simulink model "velo_pi"  (Simulink 7.9)
settings: Solver=ode4  StartTime=0.0  StopTime=20  RelTol=1e-3
values from neighbouring files (symbols this model uses):
  ts = 1/50    (= 0.02)    [velo_id_gain.m]    (also in velo_id_tc.m; velo_pi_mbd.m)
libraries: arduino_io_lib x5, simulink x1
settings Model: Creator=hirata  LastModifiedBy=hirata

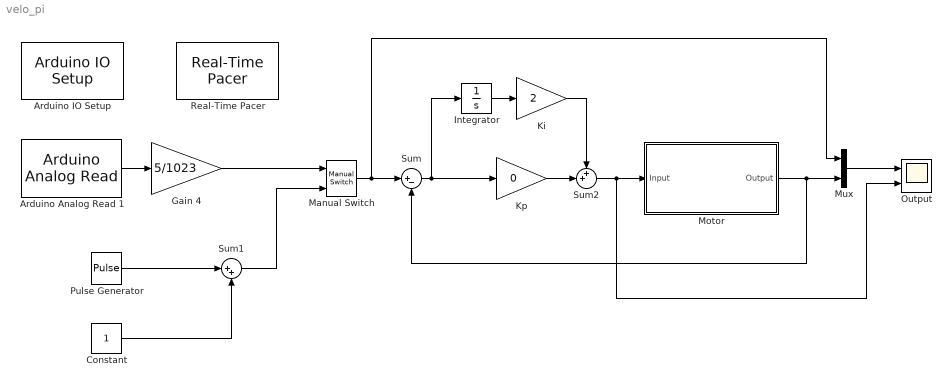
== system velo_pi ==
  Arduino Analog Read 1 : arduino_io_lib/Arduino Analog Read  arduinoVar=Temporary arduino variable: Arduino1  arduinoPin=1  T=ts
  Arduino IO Setup : arduino_io_lib/Arduino IO Setup  Priority=3  arduinoVar=Temporary arduino variable: Arduino1  workspaceVarName=a  comPort=COM3
  Constant : Constant
  Gain 4 : Gain  Gain=5/1023
  Integrator : Integrator
  Ki : Gain  Gain=2
  Kp : Gain  Gain=0
  Manual Switch : simulink/Signal Routing/Manual Switch  sw=0  action=0  varsize=off
  Motor : Subsystem
  Mux : Mux  Inputs=2
  Output : Scope  NumInputPorts=2
      settings: TimeRange=10  YMin=0~0  YMax=2~5
  Pulse Generator : DiscretePulseGenerator  Amplitude=0.5  Period=10/ts  PulseWidth=5/ts  SampleTime=ts
  Real-Time Pacer : arduino_io_lib/Real-Time Pacer  simTimePerRealTime=1
  Sum : Sum  Inputs=|+-
  Sum1 : Sum  Inputs=|++
  Sum2 : Sum  Inputs=++|
  wires:
  Motor/1(Output) -> Mux/2, Sum/2
  Mux/1 -> Output/1
  Arduino Analog Read 1/1 -> Gain 4/1
  Sum2/1 -> Motor/1(Input), Output/2
  Sum/1 -> Kp/1, Integrator/1
  Manual Switch/1 -> Sum/1, Mux/1
  Gain 4/1 -> Manual Switch/1
  Constant/1 -> Sum1/2
  Pulse Generator/1 -> Sum1/1
  Sum1/1 -> Manual Switch/2
  Integrator/1 -> Ki/1
  Ki/1 -> Sum2/1
  Kp/1 -> Sum2/2

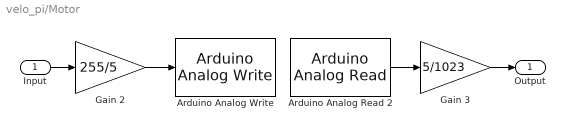
== system velo_pi/Motor ==
  Input : Inport
  Arduino Analog Read 2 : arduino_io_lib/Arduino Analog Read  arduinoVar=Temporary arduino variable: Arduino1  arduinoPin=0  T=ts
  Arduino Analog Write : arduino_io_lib/Arduino Analog Write  arduinoVar=Temporary arduino variable: Arduino1  arduinoPin=3  T=ts
  Gain 2 : Gain  Gain=255/5
  Gain 3 : Gain  Gain=5/1023
  Output : Outport
  wires:
  Arduino Analog Read 2/1 -> Gain 3/1
  Gain 2/1 -> Arduino Analog Write/1
  Input/1 -> Gain 2/1
  Gain 3/1 -> Output/1
